simulink model "Nexonar_Navigation"  (R2018b)
settings: Solver=FixedStepDiscrete  StartTime=0.0  StopTime=0.1  RelTol=1e-3  EnableMultiTasking=on
libraries: commutil2 x12, c2833xlib x5, c280xlib x5, simulink x1, c2000lib x1
(part 1 of 2)
settings Model: ExtModeTrigDuration=8  Creator=User  LastModifiedBy=hengw
settings DataIOCC: LimitDataPoints=on  SaveFormat=Array  SaveOutput=off  SaveTime=off
settings OptimizationCC: DefaultUnderspecifiedDataType=single  ExpressionDepthLimit=2147483647  LifeSpan=1  MaxStackSize=512
settings DebuggingCC: UnderspecifiedInitializationDetection=Classic  MergeDetectMultiDrivingBlocksExec=none  SolverPrmCheckMsg=warning  StateNameClashWarn=warning  SFUnexpectedBacktrackingDiag=warning  SFNoUnconditionalDefaultTransitionDiag=warning  SFExecutionAtInitializationDiag=none
settings HardwareCC: ProdBitPerChar=16  ProdBitPerInt=16  ProdBitPerPointer=32  ProdBitPerSizeT=32  ProdBitPerPtrDiffT=32  ProdLargestAtomicInteger=Integer  ProdLargestAtomicFloat=None  ProdWordSize=16  ProdLongLongMode=on  ProdHWDeviceType=Texas Instruments->C2000  TargetBitPerChar=16  TargetBitPerInt=16  TargetLargestAtomicInteger=Integer  TargetIntDivRoundTo=Zero  TargetEndianess=LittleEndian  TargetWordSize=16  TargetHWDeviceType=Texas Instruments->C2000  ProdEqTarget=off
settings ModelReferenceCC: PropagateSignalLabelsOutOfModel=off
settings SFSimCC: SimCustomSourceCode="#include \"i2c_reset.c\""  SimCustomHeaderCode="#include \"i2c_reset.h\""  SimUseLocalCustomCode=off  MATLABDynamicMemAlloc=off
settings RTWCC: SystemTargetFile=ert.tlc  HardwareBoard=TI Delfino F2833x  TemplateMakefile=ert_default_tmf  RTWUseLocalCustomCode=off  RTWUseSimCustomCode=on  CustomSourceCode="#include \"i2c_reset.c\""  CustomHeaderCode="#include \"i2c_reset.h\""  Toolchain=Texas Instruments Code Composer Studio (C2000)
settings CodeAppCC: IgnoreCustomStorageClasses=off  CustomSymbolStrType=$N$R$M  StateflowObjectComments=on  InternalIdentifier=Classic
settings ERTTargetCC: CodeReplacementLibrary=TI C28x  MultiwordLength=2048  ParMdlRefBuildCompliant=off  CPPClassGenCompliant=off  ConvertIfToSwitch=off  SuppressUnreachableDefaultCases=off
settings ConfigComp: CovMetricSettings=dw  CovHtmlReporting=on  CovSaveCumulativeToWorkspaceVar=on  CovSaveSingleToWorkspaceVar=on  CovExternalEMLEnable=off  PSAutoStubLUT=on

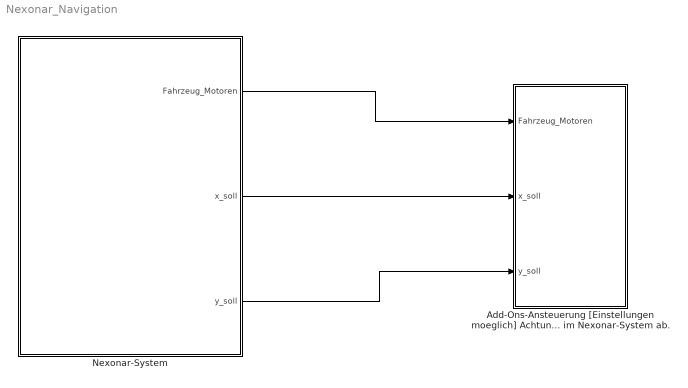
== system Nexonar_Navigation ==
  Add-Ons-Ansteuerung [Einstellungen moeglich] Achtung! Einige Einstellungswerte haengen von den Werten im Nexonar-System ab. : Subsystem
  Nexonar-System : Subsystem
  wires:
  Nexonar-System/2(x_soll) -> Add-Ons-Ansteuerung [Einstellungen moeglich] Achtung! Einige Einstellungswerte haengen von den Werten im Nexonar-System ab./2(x_soll)
  Nexonar-System/3(y_soll) -> Add-Ons-Ansteuerung [Einstellungen moeglich] Achtung! Einige Einstellungswerte haengen von den Werten im Nexonar-System ab./3(y_soll)
  Nexonar-System/1(Fahrzeug_Motoren) -> Add-Ons-Ansteuerung [Einstellungen moeglich] Achtung! Einige Einstellungswerte haengen von den Werten im Nexonar-System ab./1(Fahrzeug_Motoren)

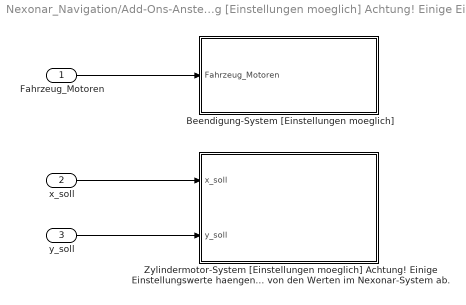
== system Nexonar_Navigation/Add-Ons-Ansteuerung [Einstellungen moeglich] Achtung! Einige Einstellungswerte haengen von den Werten im Nexonar-System ab. ==
  Fahrzeug_Motoren : Inport
  x_soll : Inport  Port=2
  y_soll : Inport  Port=3
  Beendigung-System [Einstellungen moeglich] : Subsystem
  Zylindermotor-System [Einstellungen moeglich] Achtung! Einige Einstellungswerte haengen von den Werten im Nexonar-System ab. : Subsystem
  wires:
  x_soll/1 -> Zylindermotor-System [Einstellungen moeglich] Achtung! Einige Einstellungswerte haengen von den Werten im Nexonar-System ab./1(x_soll)
  y_soll/1 -> Zylindermotor-System [Einstellungen moeglich] Achtung! Einige Einstellungswerte haengen von den Werten im Nexonar-System ab./2(y_soll)
  Fahrzeug_Motoren/1 -> Beendigung-System [Einstellungen moeglich]/1(Fahrzeug_Motoren)

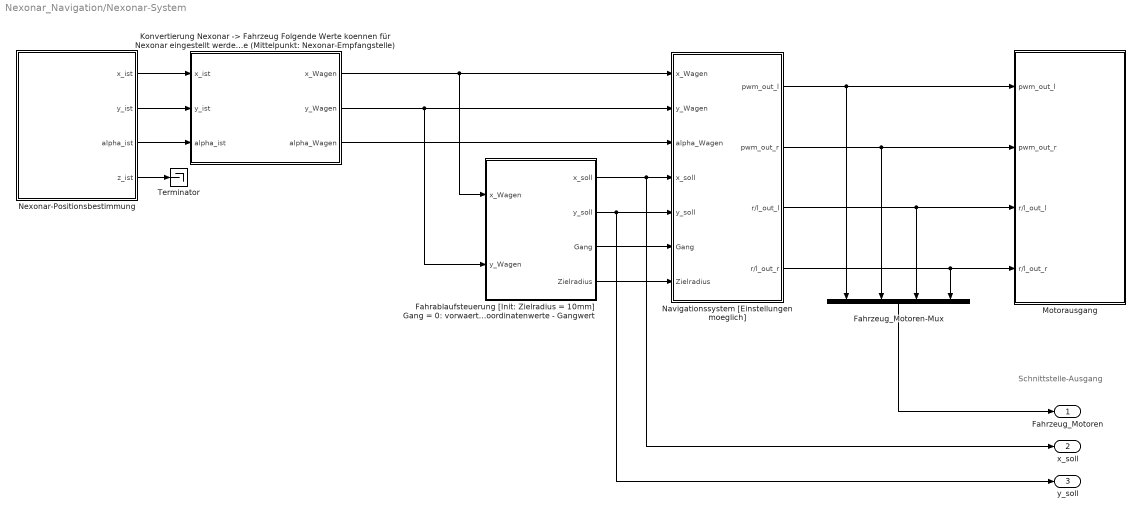
== system Nexonar_Navigation/Nexonar-System ==
  note: Schnittstelle-Ausgang
  Fahrablaufsteuerung [Init: Zielradius = 10mm] Gang = 0: vorwaerts Gang = 1: rueckwaerts Folgende Werte fuer den Ablauf sind einstellbar: - Zielkoordinatenwerte - Gangwert : Stateflow chart  TreatAsAtomicUnit=on
  Fahrzeug_Motoren-Mux : Mux
  "Konvertierung Nexonar -> Fahrzeug Folgende Werte koennen für Nexonar eingestellt werden: - r_Versatz_Nexo: Radialer Versatz des Nexonars zur Rotationsachse des Fahrzeugs - phi_Versatz_Nexo: Winkelversatz des Nexonars gegenüber der x-Achse (Mittelpunkt: Rotationspunkt des Fahrzeugs) - psi_Offset_Nexo: Winkelversatz des Nexonars gegenüber der x-Achse (Mittelpunkt: Nexonar-Empfangstelle)" : MATLAB Function  TreatAsAtomicUnit=on
  Motorausgang : Subsystem
  Navigationssystem [Einstellungen moeglich] : Subsystem  TreatAsAtomicUnit=on
  Nexonar-Positionsbestimmung : Subsystem
  Terminator : Terminator
  Fahrzeug_Motoren : Outport
  x_soll : Outport  Port=2
  y_soll : Outport  Port=3
  wires:
  Navigationssystem [Einstellungen moeglich]/3(r/l_out_l) -> Motorausgang/3(r/l_out_l), Fahrzeug_Motoren-Mux/3
  "Konvertierung Nexonar -> Fahrzeug Folgende Werte koennen für Nexonar eingestellt werden: - r_Versatz_Nexo: Radialer Versatz des Nexonars zur Rotationsachse des Fahrzeugs - phi_Versatz_Nexo: Winkelversatz des Nexonars gegenüber der x-Achse (Mittelpunkt: Rotationspunkt des Fahrzeugs) - psi_Offset_Nexo: Winkelversatz des Nexonars gegenüber der x-Achse (Mittelpunkt: Nexonar-Empfangstelle)"/2(y_Wagen) -> Fahrablaufsteuerung [Init: Zielradius = 10mm] Gang = 0: vorwaerts Gang = 1: rueckwaerts Folgende Werte fuer den Ablauf sind einstellbar: - Zielkoordinatenwerte - Gangwert/2(y_Wagen), Navigationssystem [Einstellungen moeglich]/2(y_Wagen)
  "Konvertierung Nexonar -> Fahrzeug Folgende Werte koennen für Nexonar eingestellt werden: - r_Versatz_Nexo: Radialer Versatz des Nexonars zur Rotationsachse des Fahrzeugs - phi_Versatz_Nexo: Winkelversatz des Nexonars gegenüber der x-Achse (Mittelpunkt: Rotationspunkt des Fahrzeugs) - psi_Offset_Nexo: Winkelversatz des Nexonars gegenüber der x-Achse (Mittelpunkt: Nexonar-Empfangstelle)"/1(x_Wagen) -> Fahrablaufsteuerung [Init: Zielradius = 10mm] Gang = 0: vorwaerts Gang = 1: rueckwaerts Folgende Werte fuer den Ablauf sind einstellbar: - Zielkoordinatenwerte - Gangwert/1(x_Wagen), Navigationssystem [Einstellungen moeglich]/1(x_Wagen)
  Nexonar-Positionsbestimmung/4(z_ist) -> Terminator/1
  Nexonar-Positionsbestimmung/1(x_ist) -> "Konvertierung Nexonar -> Fahrzeug Folgende Werte koennen für Nexonar eingestellt werden: - r_Versatz_Nexo: Radialer Versatz des Nexonars zur Rotationsachse des Fahrzeugs - phi_Versatz_Nexo: Winkelversatz des Nexonars gegenüber der x-Achse (Mittelpunkt: Rotationspunkt des Fahrzeugs) - psi_Offset_Nexo: Winkelversatz des Nexonars gegenüber der x-Achse (Mittelpunkt: Nexonar-Empfangstelle)"/1(x_ist)
  Fahrablaufsteuerung [Init: Zielradius = 10mm] Gang = 0: vorwaerts Gang = 1: rueckwaerts Folgende Werte fuer den Ablauf sind einstellbar: - Zielkoordinatenwerte - Gangwert/2(y_soll) -> y_soll/1, Navigationssystem [Einstellungen moeglich]/5(y_soll)
  Fahrablaufsteuerung [Init: Zielradius = 10mm] Gang = 0: vorwaerts Gang = 1: rueckwaerts Folgende Werte fuer den Ablauf sind einstellbar: - Zielkoordinatenwerte - Gangwert/1(x_soll) -> x_soll/1, Navigationssystem [Einstellungen moeglich]/4(x_soll)
  Navigationssystem [Einstellungen moeglich]/4(r/l_out_r) -> Motorausgang/4(r/l_out_r), Fahrzeug_Motoren-Mux/4
  Nexonar-Positionsbestimmung/3(alpha_ist) -> "Konvertierung Nexonar -> Fahrzeug Folgende Werte koennen für Nexonar eingestellt werden: - r_Versatz_Nexo: Radialer Versatz des Nexonars zur Rotationsachse des Fahrzeugs - phi_Versatz_Nexo: Winkelversatz des Nexonars gegenüber der x-Achse (Mittelpunkt: Rotationspunkt des Fahrzeugs) - psi_Offset_Nexo: Winkelversatz des Nexonars gegenüber der x-Achse (Mittelpunkt: Nexonar-Empfangstelle)"/3(alpha_ist)
  "Konvertierung Nexonar -> Fahrzeug Folgende Werte koennen für Nexonar eingestellt werden: - r_Versatz_Nexo: Radialer Versatz des Nexonars zur Rotationsachse des Fahrzeugs - phi_Versatz_Nexo: Winkelversatz des Nexonars gegenüber der x-Achse (Mittelpunkt: Rotationspunkt des Fahrzeugs) - psi_Offset_Nexo: Winkelversatz des Nexonars gegenüber der x-Achse (Mittelpunkt: Nexonar-Empfangstelle)"/3(alpha_Wagen) -> Navigationssystem [Einstellungen moeglich]/3(alpha_Wagen)
  Fahrablaufsteuerung [Init: Zielradius = 10mm] Gang = 0: vorwaerts Gang = 1: rueckwaerts Folgende Werte fuer den Ablauf sind einstellbar: - Zielkoordinatenwerte - Gangwert/3(Gang) -> Navigationssystem [Einstellungen moeglich]/6(Gang)
  Fahrablaufsteuerung [Init: Zielradius = 10mm] Gang = 0: vorwaerts Gang = 1: rueckwaerts Folgende Werte fuer den Ablauf sind einstellbar: - Zielkoordinatenwerte - Gangwert/4(Zielradius) -> Navigationssystem [Einstellungen moeglich]/7(Zielradius)
  Nexonar-Positionsbestimmung/2(y_ist) -> "Konvertierung Nexonar -> Fahrzeug Folgende Werte koennen für Nexonar eingestellt werden: - r_Versatz_Nexo: Radialer Versatz des Nexonars zur Rotationsachse des Fahrzeugs - phi_Versatz_Nexo: Winkelversatz des Nexonars gegenüber der x-Achse (Mittelpunkt: Rotationspunkt des Fahrzeugs) - psi_Offset_Nexo: Winkelversatz des Nexonars gegenüber der x-Achse (Mittelpunkt: Nexonar-Empfangstelle)"/2(y_ist)
  Fahrzeug_Motoren-Mux/1 -> Fahrzeug_Motoren/1
  Navigationssystem [Einstellungen moeglich]/1(pwm_out_l) -> Motorausgang/1(pwm_out_l), Fahrzeug_Motoren-Mux/1
  Navigationssystem [Einstellungen moeglich]/2(pwm_out_r) -> Motorausgang/2(pwm_out_r), Fahrzeug_Motoren-Mux/2

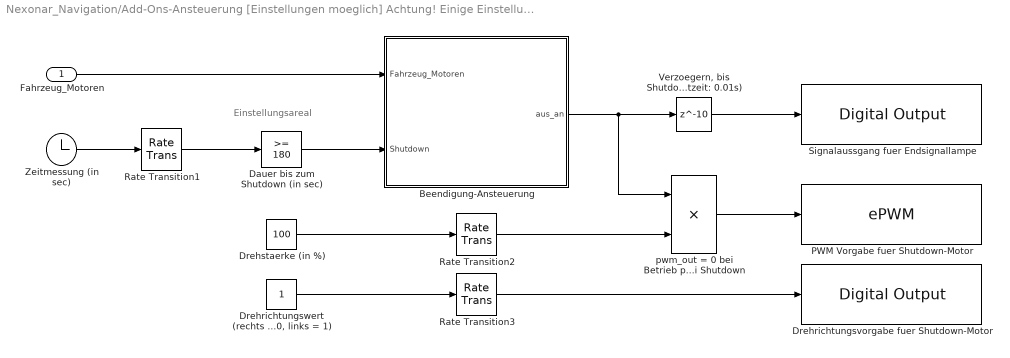
== system Nexonar_Navigation/Add-Ons-Ansteuerung [Einstellungen moeglich] Achtung! Einige Einstellungswerte haengen von den Werten im Nexonar-System ab./Beendigung-System [Einstellungen moeglich] ==
  note: Einstellungsareal
  Fahrzeug_Motoren : Inport
  Beendigung-Ansteuerung : Stateflow chart  TreatAsAtomicUnit=on
  Dauer bis zum Shutdown (in sec) : simulink/Logic and Bit Operations/Compare To Constant  relop=>=  const=180  OutDataTypeStr=boolean
  Drehrichtungsvorgabe fuer Shutdown-Motor : c2833xlib/Digital Output  GPIO_Number=GPIO8~GPIO15  GPIO_Bit0=off  GPIO_BIT0_Toggle=off  GPIO_Bit1=off  GPIO_BIT1_Toggle=off  GPIO_Bit2=off  GPIO_BIT2_Toggle=off  GPIO_Bit3=off  GPIO_BIT3_Toggle=off  GPIO_Bit4=off  GPIO_BIT4_Toggle=off  GPIO_Bit5=off  GPIO_BIT5_Toggle=off  GPIO_Bit6=off  GPIO_BIT6_Toggle=off  GPIO_Bit7=on  GPIO_BIT7_Toggle=off
      settings: SourceProductName=Embedded Coder Support Package for Texas Instruments C2000 Processors  SourceProductBaseCode=TIC2000
  "Drehrichtungswert (rechts = 0, links = 1)" : Constant
  Drehstaerke (in %) : Constant  Value=100
  "PWM Vorgabe fuer Shutdown-Motor " : c280xlib/ePWM  checkMode=off  useModule=ePWM5  periodUnits=Clock cycles  timerSource=Specify via dialog  timerPeriod_clk=64000  timerPeriod_sec=0.0001  tbshadow=Counter equals to zero  countingMode=Up  phaseActiveEnable=Disable  phaseDirection=Count down after sync  phaseActive=0  synchronizationEnable=off  synchronizationOption=Disable  clockPrescale=1  HSclockPrescale=1  ePWMxAStatus=off  CMPAUnits=Clock cycles  CMPASource=Specify via dialog  CMPAValue_per=50  CMPAValue_clk=32000  enCMPAshadow=Counter equals to zero  ePWMxAactionLogic1=Do nothing  ePWMxAactionLogic2=Clear  ePWMxAactionLogic3=Set  ePWMxAactionLogic4=Do nothing  ePWMxAactionLogic5=Do nothing  ePWMxAactionLogic6=Do nothing  ePWMxALoadMode=Load on counter equals to zero (CTR=Zero)  ePWMxACSFenable=off  ePWMxACSFvalue=Forcing disable  ePWMxASFreload=Zero  enHRPWM=off  HRPWM_LoadMode=Counter equals to zero (CTR=ZERO)  HRPWM_CTLMode=Phase control mode  HRPWM_EDGMode=Both edge  enSFO=on  ePWMxBStatus=on  CMPBUnits=Percentages  CMPBSource=Input port  CMPBValue_per=0  CMPBValue_clk=32000  enCMPBshadow=Counter equals to zero  ePWMxBactionLogic1=Do nothing  ePWMxBactionLogic2=Set  ePWMxBactionLogic3=Do nothing  ePWMxBactionLogic4=Do nothing  ePWMxBactionLogic5=Clear  ePWMxBactionLogic6=Do nothing  ePWMxBLoadMode=Load on counter equals to zero (CTR=Zero)  ePWMxBCSFenable=off  ePWMxBCSFvalue=Forcing disable  ePWMxBSFreload=Zero  enableDBePWMxA=off  enableDBePWMxB=off  DBpolarity=Active high (AH)  DBedgeDelay=Positive  DBSource_ePWMxA=ePWMxA  DBSource_ePWMxB=ePWMxA  DBperiodSource=Specify via dialog  REDperiod=0  FEDperiod=0  adcstartModuleA=off  adcrequestEventA=First event  adcstartEventA=Counter equals to zero (CTR=Zero)  adcstartModuleB=off  adcrequestEventB=First event  adcstartEventB=Counter equals to zero (CTR=Zero)  intEn=off  intPrd=First event  intSel=Counter equals to zero (CTR=Zero)  chopperEnable=off  chopperFrequency=1  chopperFirstwidth=1  chopperDuty=12.5%  tripZonesource=Specify via dialog  tzselOSHT1=off  tzselOSHT2=off  tzselOSHT3=off  tzselOSHT4=off  tzselOSHT5=off  tzselOSHT6=off  tzselCBC1=off  tzselCBC2=off  tzselCBC3=off  tzselCBC4=off  tzselCBC5=off  tzselCBC6=off  enTzOstIntr=off  enTzCbcIntr=off  ePWMxAforced=No action  ePWMxBforced=No action  timerPeriod=-1  ePWMxAValue=0  ePWMxBValue=0  tripZoneoption=One-shot trip (OSHT)
      settings: SourceProductName=Embedded Coder Support Package for Texas Instruments C2000 Processors  SourceProductBaseCode=TIC2000
  Rate Transition1 : RateTransition  OutPortSampleTime=0.01
  Rate Transition2 : RateTransition  OutPortSampleTime=0.01
  Rate Transition3 : RateTransition  OutPortSampleTime=0.01
  Signalaussgang fuer Endsignallampe : c2833xlib/Digital Output  GPIO_Number=GPIO56~GPIO63  GPIO_Bit0=off  GPIO_BIT0_Toggle=off  GPIO_Bit1=off  GPIO_BIT1_Toggle=off  GPIO_Bit2=on  GPIO_BIT2_Toggle=off  GPIO_Bit3=off  GPIO_BIT3_Toggle=off  GPIO_Bit4=off  GPIO_BIT4_Toggle=off  GPIO_Bit5=off  GPIO_BIT5_Toggle=off  GPIO_Bit6=off  GPIO_BIT6_Toggle=off  GPIO_Bit7=off  GPIO_BIT7_Toggle=off
      settings: SourceProductName=Embedded Coder Support Package for Texas Instruments C2000 Processors  SourceProductBaseCode=TIC2000
  "Verzoegern, bis Shutdown ausgefuehrt ist (Abtastzeit: 0.01s)" : Delay  DelayLength=10  InitialCondition=0
  Zeitmessung (in sec) : Clock
  pwm_out = 0 bei Betrieb pwm_out = Drehstaerke bei Shutdown : Product
  wires:
  Zeitmessung (in sec)/1 -> Rate Transition1/1
  pwm_out = 0 bei Betrieb pwm_out = Drehstaerke bei Shutdown/1 -> "PWM Vorgabe fuer Shutdown-Motor "/1
  "Drehrichtungswert (rechts = 0, links = 1)"/1 -> Rate Transition3/1
  Fahrzeug_Motoren/1 -> Beendigung-Ansteuerung/1(Fahrzeug_Motoren)
  Beendigung-Ansteuerung/1(aus_an) -> pwm_out = 0 bei Betrieb pwm_out = Drehstaerke bei Shutdown/1, "Verzoegern, bis Shutdown ausgefuehrt ist (Abtastzeit: 0.01s)"/1
  "Verzoegern, bis Shutdown ausgefuehrt ist (Abtastzeit: 0.01s)"/1 -> Signalaussgang fuer Endsignallampe/1
  Rate Transition3/1 -> Drehrichtungsvorgabe fuer Shutdown-Motor/1
  Dauer bis zum Shutdown (in sec)/1 -> Beendigung-Ansteuerung/2(Shutdown)
  Drehstaerke (in %)/1 -> Rate Transition2/1
  Rate Transition2/1 -> pwm_out = 0 bei Betrieb pwm_out = Drehstaerke bei Shutdown/2
  Rate Transition1/1 -> Dauer bis zum Shutdown (in sec)/1

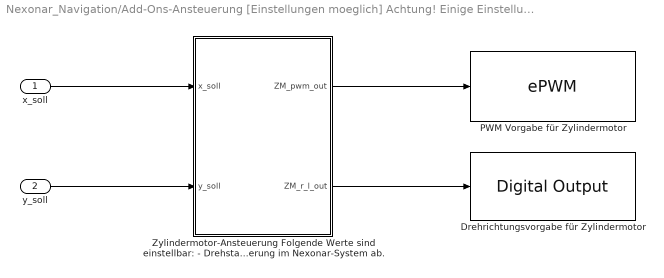
== system Nexonar_Navigation/Add-Ons-Ansteuerung [Einstellungen moeglich] Achtung! Einige Einstellungswerte haengen von den Werten im Nexonar-System ab./Zylindermotor-System [Einstellungen moeglich] Achtung! Einige Einstellungswerte haengen von den Werten im Nexonar-System ab. ==
  x_soll : Inport
  y_soll : Inport  Port=2
  Drehrichtungsvorgabe für Zylindermotor : c2833xlib/Digital Output  GPIO_Number=GPIO16~GPIO23  GPIO_Bit0=off  GPIO_BIT0_Toggle=off  GPIO_Bit1=on  GPIO_BIT1_Toggle=off  GPIO_Bit2=off  GPIO_BIT2_Toggle=off  GPIO_Bit3=off  GPIO_BIT3_Toggle=off  GPIO_Bit4=off  GPIO_BIT4_Toggle=off  GPIO_Bit5=off  GPIO_BIT5_Toggle=off  GPIO_Bit6=off  GPIO_BIT6_Toggle=off  GPIO_Bit7=off  GPIO_BIT7_Toggle=off
      settings: SourceProductName=Embedded Coder Support Package for Texas Instruments C2000 Processors  SourceProductBaseCode=TIC2000
  PWM Vorgabe für Zylindermotor : c280xlib/ePWM  checkMode=off  useModule=ePWM3  periodUnits=Clock cycles  timerSource=Specify via dialog  timerPeriod_clk=64000  timerPeriod_sec=0.0001  tbshadow=Counter equals to zero  countingMode=Up  phaseActiveEnable=Disable  phaseDirection=Count down after sync  phaseActive=0  synchronizationEnable=off  synchronizationOption=Disable  clockPrescale=1  HSclockPrescale=1  ePWMxAStatus=off  CMPAUnits=Clock cycles  CMPASource=Specify via dialog  CMPAValue_per=50  CMPAValue_clk=32000  enCMPAshadow=Counter equals to zero  ePWMxAactionLogic1=Do nothing  ePWMxAactionLogic2=Clear  ePWMxAactionLogic3=Set  ePWMxAactionLogic4=Do nothing  ePWMxAactionLogic5=Do nothing  ePWMxAactionLogic6=Do nothing  ePWMxALoadMode=Load on counter equals to zero (CTR=Zero)  ePWMxACSFenable=off  ePWMxACSFvalue=Forcing disable  ePWMxASFreload=Zero  enHRPWM=off  HRPWM_LoadMode=Counter equals to zero (CTR=ZERO)  HRPWM_CTLMode=Phase control mode  HRPWM_EDGMode=Both edge  enSFO=on  ePWMxBStatus=on  CMPBUnits=Percentages  CMPBSource=Input port  CMPBValue_per=0  CMPBValue_clk=32000  enCMPBshadow=Counter equals to zero  ePWMxBactionLogic1=Do nothing  ePWMxBactionLogic2=Set  ePWMxBactionLogic3=Do nothing  ePWMxBactionLogic4=Do nothing  ePWMxBactionLogic5=Clear  ePWMxBactionLogic6=Do nothing  ePWMxBLoadMode=Load on counter equals to zero (CTR=Zero)  ePWMxBCSFenable=off  ePWMxBCSFvalue=Forcing disable  ePWMxBSFreload=Zero  enableDBePWMxA=off  enableDBePWMxB=off  DBpolarity=Active high (AH)  DBedgeDelay=Positive  DBSource_ePWMxA=ePWMxA  DBSource_ePWMxB=ePWMxA  DBperiodSource=Specify via dialog  REDperiod=0  FEDperiod=0  adcstartModuleA=off  adcrequestEventA=First event  adcstartEventA=Counter equals to zero (CTR=Zero)  adcstartModuleB=off  adcrequestEventB=First event  adcstartEventB=Counter equals to zero (CTR=Zero)  intEn=off  intPrd=First event  intSel=Counter equals to zero (CTR=Zero)  chopperEnable=off  chopperFrequency=1  chopperFirstwidth=1  chopperDuty=12.5%  tripZonesource=Specify via dialog  tzselOSHT1=off  tzselOSHT2=off  tzselOSHT3=off  tzselOSHT4=off  tzselOSHT5=off  tzselOSHT6=off  tzselCBC1=off  tzselCBC2=off  tzselCBC3=off  tzselCBC4=off  tzselCBC5=off  tzselCBC6=off  enTzOstIntr=off  enTzCbcIntr=off  ePWMxAforced=No action  ePWMxBforced=No action  timerPeriod=-1  ePWMxAValue=0  ePWMxBValue=0  tripZoneoption=One-shot trip (OSHT)
      settings: SourceProductName=Embedded Coder Support Package for Texas Instruments C2000 Processors  SourceProductBaseCode=TIC2000
  "Zylindermotor-Ansteuerung Folgende Werte sind einstellbar: - Drehstaerke (in %) (-> ZM_pwm_out in \"Ausfuerung\") - Drehrichtung (rechts = 0, links = 1) (-> ZM_r_l_out in \"Init_und_Warten\") - Drehdauer (-> zwischen \"Ausfuehrung\" und \"Beendet\") - Ausfuehrungspunkt (in mm) [durch Wechsel der Soll-Position] (-> zwischen \"Init_und_Start\" und \"Ausfuehrung) Wichtig! Der Ausfuerungspunkt haengt von den EXAKTEN Soll-Werten aus der Fahrablaufsteuerung im Nexonar-System ab." : Stateflow chart  TreatAsAtomicUnit=on
  wires:
  "Zylindermotor-Ansteuerung Folgende Werte sind einstellbar: - Drehstaerke (in %) (-> ZM_pwm_out in \"Ausfuerung\") - Drehrichtung (rechts = 0, links = 1) (-> ZM_r_l_out in \"Init_und_Warten\") - Drehdauer (-> zwischen \"Ausfuehrung\" und \"Beendet\") - Ausfuehrungspunkt (in mm) [durch Wechsel der Soll-Position] (-> zwischen \"Init_und_Start\" und \"Ausfuehrung) Wichtig! Der Ausfuerungspunkt haengt von den EXAKTEN Soll-Werten aus der Fahrablaufsteuerung im Nexonar-System ab."/1(ZM_pwm_out) -> PWM Vorgabe für Zylindermotor/1
  "Zylindermotor-Ansteuerung Folgende Werte sind einstellbar: - Drehstaerke (in %) (-> ZM_pwm_out in \"Ausfuerung\") - Drehrichtung (rechts = 0, links = 1) (-> ZM_r_l_out in \"Init_und_Warten\") - Drehdauer (-> zwischen \"Ausfuehrung\" und \"Beendet\") - Ausfuehrungspunkt (in mm) [durch Wechsel der Soll-Position] (-> zwischen \"Init_und_Start\" und \"Ausfuehrung) Wichtig! Der Ausfuerungspunkt haengt von den EXAKTEN Soll-Werten aus der Fahrablaufsteuerung im Nexonar-System ab."/2(ZM_r_l_out) -> Drehrichtungsvorgabe für Zylindermotor/1
  y_soll/1 -> "Zylindermotor-Ansteuerung Folgende Werte sind einstellbar: - Drehstaerke (in %) (-> ZM_pwm_out in \"Ausfuerung\") - Drehrichtung (rechts = 0, links = 1) (-> ZM_r_l_out in \"Init_und_Warten\") - Drehdauer (-> zwischen \"Ausfuehrung\" und \"Beendet\") - Ausfuehrungspunkt (in mm) [durch Wechsel der Soll-Position] (-> zwischen \"Init_und_Start\" und \"Ausfuehrung) Wichtig! Der Ausfuerungspunkt haengt von den EXAKTEN Soll-Werten aus der Fahrablaufsteuerung im Nexonar-System ab."/2(y_soll)
  x_soll/1 -> "Zylindermotor-Ansteuerung Folgende Werte sind einstellbar: - Drehstaerke (in %) (-> ZM_pwm_out in \"Ausfuerung\") - Drehrichtung (rechts = 0, links = 1) (-> ZM_r_l_out in \"Init_und_Warten\") - Drehdauer (-> zwischen \"Ausfuehrung\" und \"Beendet\") - Ausfuehrungspunkt (in mm) [durch Wechsel der Soll-Position] (-> zwischen \"Init_und_Start\" und \"Ausfuehrung) Wichtig! Der Ausfuerungspunkt haengt von den EXAKTEN Soll-Werten aus der Fahrablaufsteuerung im Nexonar-System ab."/1(x_soll)

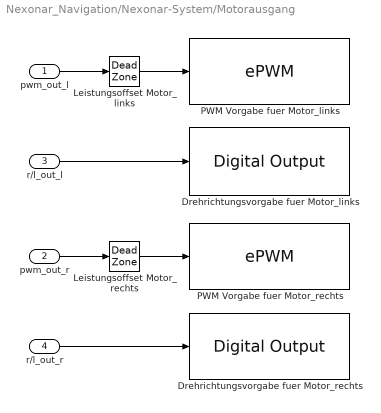
== system Nexonar_Navigation/Nexonar-System/Motorausgang ==
  pwm_out_l : Inport
  pwm_out_r : Inport  Port=2
  r/l_out_l : Inport  Port=3
  r/l_out_r : Inport  Port=4
  Drehrichtungsvorgabe fuer Motor_links : c2833xlib/Digital Output  GPIO_Number=GPIO16~GPIO23  GPIO_Bit0=off  GPIO_BIT0_Toggle=off  GPIO_Bit1=off  GPIO_BIT1_Toggle=off  GPIO_Bit2=off  GPIO_BIT2_Toggle=off  GPIO_Bit3=off  GPIO_BIT3_Toggle=off  GPIO_Bit4=on  GPIO_BIT4_Toggle=off  GPIO_Bit5=off  GPIO_BIT5_Toggle=off  GPIO_Bit6=off  GPIO_BIT6_Toggle=off  GPIO_Bit7=off  GPIO_BIT7_Toggle=off
      settings: SourceProductName=Embedded Coder Support Package for Texas Instruments C2000 Processors  SourceProductBaseCode=TIC2000
  Drehrichtungsvorgabe fuer Motor_rechts : c2833xlib/Digital Output  GPIO_Number=GPIO16~GPIO23  GPIO_Bit0=off  GPIO_BIT0_Toggle=off  GPIO_Bit1=off  GPIO_BIT1_Toggle=off  GPIO_Bit2=off  GPIO_BIT2_Toggle=off  GPIO_Bit3=off  GPIO_BIT3_Toggle=off  GPIO_Bit4=off  GPIO_BIT4_Toggle=off  GPIO_Bit5=on  GPIO_BIT5_Toggle=off  GPIO_Bit6=off  GPIO_BIT6_Toggle=off  GPIO_Bit7=off  GPIO_BIT7_Toggle=off
      settings: SourceProductName=Embedded Coder Support Package for Texas Instruments C2000 Processors  SourceProductBaseCode=TIC2000
  Leistungsoffset Motor_links : DeadZone  LowerValue=0  UpperValue=0  SaturateOnIntegerOverflow=on
  Leistungsoffset Motor_rechts : DeadZone  LowerValue=0  UpperValue=5  SaturateOnIntegerOverflow=on
  "PWM Vorgabe fuer Motor_links " : c280xlib/ePWM  checkMode=off  useModule=ePWM1  periodUnits=Clock cycles  timerSource=Specify via dialog  timerPeriod_clk=64000  timerPeriod_sec=0.0001  tbshadow=Counter equals to zero  countingMode=Up  phaseActiveEnable=Disable  phaseDirection=Count down after sync  phaseActive=0  synchronizationEnable=off  synchronizationOption=Disable  clockPrescale=1  HSclockPrescale=1  ePWMxAStatus=off  CMPAUnits=Clock cycles  CMPASource=Specify via dialog  CMPAValue_per=50  CMPAValue_clk=32000  enCMPAshadow=Counter equals to zero  ePWMxAactionLogic1=Do nothing  ePWMxAactionLogic2=Clear  ePWMxAactionLogic3=Set  ePWMxAactionLogic4=Do nothing  ePWMxAactionLogic5=Do nothing  ePWMxAactionLogic6=Do nothing  ePWMxALoadMode=Load on counter equals to zero (CTR=Zero)  ePWMxACSFenable=off  ePWMxACSFvalue=Forcing disable  ePWMxASFreload=Zero  enHRPWM=off  HRPWM_LoadMode=Counter equals to zero (CTR=ZERO)  HRPWM_CTLMode=Phase control mode  HRPWM_EDGMode=Both edge  enSFO=on  ePWMxBStatus=on  CMPBUnits=Percentages  CMPBSource=Input port  CMPBValue_per=0  CMPBValue_clk=32000  enCMPBshadow=Counter equals to zero  ePWMxBactionLogic1=Do nothing  ePWMxBactionLogic2=Set  ePWMxBactionLogic3=Do nothing  ePWMxBactionLogic4=Do nothing  ePWMxBactionLogic5=Clear  ePWMxBactionLogic6=Do nothing  ePWMxBLoadMode=Load on counter equals to zero (CTR=Zero)  ePWMxBCSFenable=off  ePWMxBCSFvalue=Forcing disable  ePWMxBSFreload=Zero  enableDBePWMxA=off  enableDBePWMxB=off  DBpolarity=Active high (AH)  DBedgeDelay=Positive  DBSource_ePWMxA=ePWMxA  DBSource_ePWMxB=ePWMxA  DBperiodSource=Specify via dialog  REDperiod=0  FEDperiod=0  adcstartModuleA=off  adcrequestEventA=First event  adcstartEventA=Counter equals to zero (CTR=Zero)  adcstartModuleB=off  adcrequestEventB=First event  adcstartEventB=Counter equals to zero (CTR=Zero)  intEn=off  intPrd=First event  intSel=Counter equals to zero (CTR=Zero)  chopperEnable=off  chopperFrequency=1  chopperFirstwidth=1  chopperDuty=12.5%  tripZonesource=Specify via dialog  tzselOSHT1=off  tzselOSHT2=off  tzselOSHT3=off  tzselOSHT4=off  tzselOSHT5=off  tzselOSHT6=off  tzselCBC1=off  tzselCBC2=off  tzselCBC3=off  tzselCBC4=off  tzselCBC5=off  tzselCBC6=off  enTzOstIntr=off  enTzCbcIntr=off  ePWMxAforced=No action  ePWMxBforced=No action  timerPeriod=-1  ePWMxAValue=0  ePWMxBValue=0  tripZoneoption=One-shot trip (OSHT)
      settings: SourceProductName=Embedded Coder Support Package for Texas Instruments C2000 Processors  SourceProductBaseCode=TIC2000
  PWM Vorgabe fuer Motor_rechts : c280xlib/ePWM  checkMode=off  useModule=ePWM2  periodUnits=Clock cycles  timerSource=Specify via dialog  timerPeriod_clk=64000  timerPeriod_sec=0.0001  tbshadow=Counter equals to zero  countingMode=Up  phaseActiveEnable=Disable  phaseDirection=Count down after sync  phaseActive=0  synchronizationEnable=off  synchronizationOption=Disable  clockPrescale=1  HSclockPrescale=1  ePWMxAStatus=off  CMPAUnits=Clock cycles  CMPASource=Specify via dialog  CMPAValue_per=50  CMPAValue_clk=32000  enCMPAshadow=Counter equals to zero  ePWMxAactionLogic1=Do nothing  ePWMxAactionLogic2=Clear  ePWMxAactionLogic3=Set  ePWMxAactionLogic4=Do nothing  ePWMxAactionLogic5=Do nothing  ePWMxAactionLogic6=Do nothing  ePWMxALoadMode=Load on counter equals to zero (CTR=Zero)  ePWMxACSFenable=off  ePWMxACSFvalue=Forcing disable  ePWMxASFreload=Zero  enHRPWM=off  HRPWM_LoadMode=Counter equals to zero (CTR=ZERO)  HRPWM_CTLMode=Phase control mode  HRPWM_EDGMode=Both edge  enSFO=on  ePWMxBStatus=on  CMPBUnits=Percentages  CMPBSource=Input port  CMPBValue_per=0  CMPBValue_clk=32000  enCMPBshadow=Counter equals to zero  ePWMxBactionLogic1=Do nothing  ePWMxBactionLogic2=Set  ePWMxBactionLogic3=Do nothing  ePWMxBactionLogic4=Do nothing  ePWMxBactionLogic5=Clear  ePWMxBactionLogic6=Do nothing  ePWMxBLoadMode=Load on counter equals to zero (CTR=Zero)  ePWMxBCSFenable=off  ePWMxBCSFvalue=Forcing disable  ePWMxBSFreload=Zero  enableDBePWMxA=off  enableDBePWMxB=off  DBpolarity=Active high (AH)  DBedgeDelay=Positive  DBSource_ePWMxA=ePWMxA  DBSource_ePWMxB=ePWMxA  DBperiodSource=Specify via dialog  REDperiod=0  FEDperiod=0  adcstartModuleA=off  adcrequestEventA=First event  adcstartEventA=Counter equals to zero (CTR=Zero)  adcstartModuleB=off  adcrequestEventB=First event  adcstartEventB=Counter equals to zero (CTR=Zero)  intEn=off  intPrd=First event  intSel=Counter equals to zero (CTR=Zero)  chopperEnable=off  chopperFrequency=1  chopperFirstwidth=1  chopperDuty=12.5%  tripZonesource=Specify via dialog  tzselOSHT1=off  tzselOSHT2=off  tzselOSHT3=off  tzselOSHT4=off  tzselOSHT5=off  tzselOSHT6=off  tzselCBC1=off  tzselCBC2=off  tzselCBC3=off  tzselCBC4=off  tzselCBC5=off  tzselCBC6=off  enTzOstIntr=off  enTzCbcIntr=off  ePWMxAforced=No action  ePWMxBforced=No action  timerPeriod=-1  ePWMxAValue=0  ePWMxBValue=0  tripZoneoption=One-shot trip (OSHT)
      settings: SourceProductName=Embedded Coder Support Package for Texas Instruments C2000 Processors  SourceProductBaseCode=TIC2000
  wires:
  pwm_out_l/1 -> Leistungsoffset Motor_links/1
  pwm_out_r/1 -> Leistungsoffset Motor_rechts/1
  r/l_out_l/1 -> Drehrichtungsvorgabe fuer Motor_links/1
  r/l_out_r/1 -> Drehrichtungsvorgabe fuer Motor_rechts/1
  Leistungsoffset Motor_links/1 -> "PWM Vorgabe fuer Motor_links "/1
  Leistungsoffset Motor_rechts/1 -> PWM Vorgabe fuer Motor_rechts/1

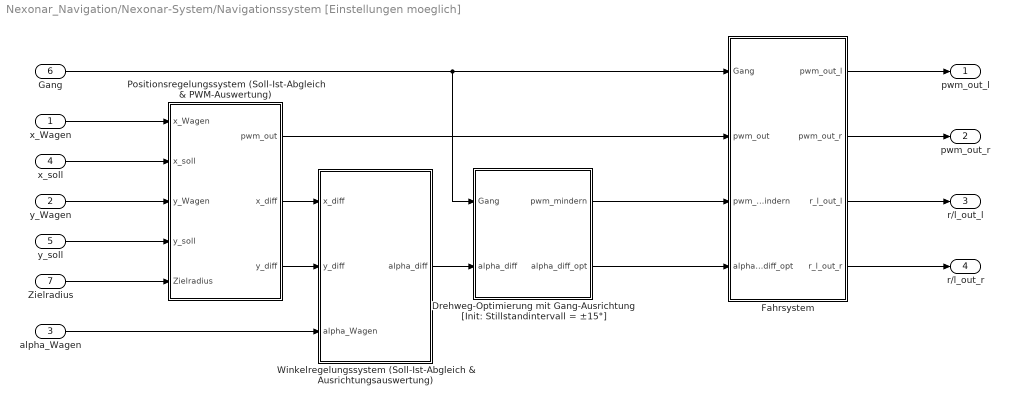
== system Nexonar_Navigation/Nexonar-System/Navigationssystem [Einstellungen moeglich] ==
  x_Wagen : Inport
  y_Wagen : Inport  Port=2
  alpha_Wagen : Inport  Port=3
  x_soll : Inport  Port=4
  y_soll : Inport  Port=5
  Gang : Inport  Port=6
  Zielradius : Inport  Port=7
  Drehweg-Optimierung mit Gang-Ausrichtung [Init: Stillstandintervall = ±15°] : Stateflow chart  TreatAsAtomicUnit=on
  Fahrsystem : Stateflow chart  TreatAsAtomicUnit=on
  Positionsregelungssystem (Soll-Ist-Abgleich & PWM-Auswertung) : Subsystem
  Winkelregelungssystem (Soll-Ist-Abgleich & Ausrichtungsauswertung) : Subsystem
  pwm_out_l : Outport
  pwm_out_r : Outport  Port=2
  r/l_out_l : Outport  Port=3
  r/l_out_r : Outport  Port=4
  wires:
  Positionsregelungssystem (Soll-Ist-Abgleich & PWM-Auswertung)/2(x_diff) -> Winkelregelungssystem (Soll-Ist-Abgleich & Ausrichtungsauswertung)/1(x_diff)
  y_soll/1 -> Positionsregelungssystem (Soll-Ist-Abgleich & PWM-Auswertung)/4(y_soll)
  y_Wagen/1 -> Positionsregelungssystem (Soll-Ist-Abgleich & PWM-Auswertung)/3(y_Wagen)
  Gang/1 -> Fahrsystem/1(Gang), Drehweg-Optimierung mit Gang-Ausrichtung [Init: Stillstandintervall = ±15°]/1(Gang)
  Positionsregelungssystem (Soll-Ist-Abgleich & PWM-Auswertung)/3(y_diff) -> Winkelregelungssystem (Soll-Ist-Abgleich & Ausrichtungsauswertung)/2(y_diff)
  x_Wagen/1 -> Positionsregelungssystem (Soll-Ist-Abgleich & PWM-Auswertung)/1(x_Wagen)
  x_soll/1 -> Positionsregelungssystem (Soll-Ist-Abgleich & PWM-Auswertung)/2(x_soll)
  alpha_Wagen/1 -> Winkelregelungssystem (Soll-Ist-Abgleich & Ausrichtungsauswertung)/3(alpha_Wagen)
  Fahrsystem/2(pwm_out_r) -> pwm_out_r/1
  Fahrsystem/4(r_l_out_r) -> r/l_out_r/1
  Fahrsystem/1(pwm_out_l) -> pwm_out_l/1
  Fahrsystem/3(r_l_out_l) -> r/l_out_l/1
  Winkelregelungssystem (Soll-Ist-Abgleich & Ausrichtungsauswertung)/1(alpha_diff) -> Drehweg-Optimierung mit Gang-Ausrichtung [Init: Stillstandintervall = ±15°]/2(alpha_diff)
  Drehweg-Optimierung mit Gang-Ausrichtung [Init: Stillstandintervall = ±15°]/2(alpha_diff_opt) -> Fahrsystem/4(alpha_diff_opt)
  Zielradius/1 -> Positionsregelungssystem (Soll-Ist-Abgleich & PWM-Auswertung)/5(Zielradius)
  Drehweg-Optimierung mit Gang-Ausrichtung [Init: Stillstandintervall = ±15°]/1(pwm_mindern) -> Fahrsystem/3(pwm_mindern)
  Positionsregelungssystem (Soll-Ist-Abgleich & PWM-Auswertung)/1(pwm_out) -> Fahrsystem/2(pwm_out)

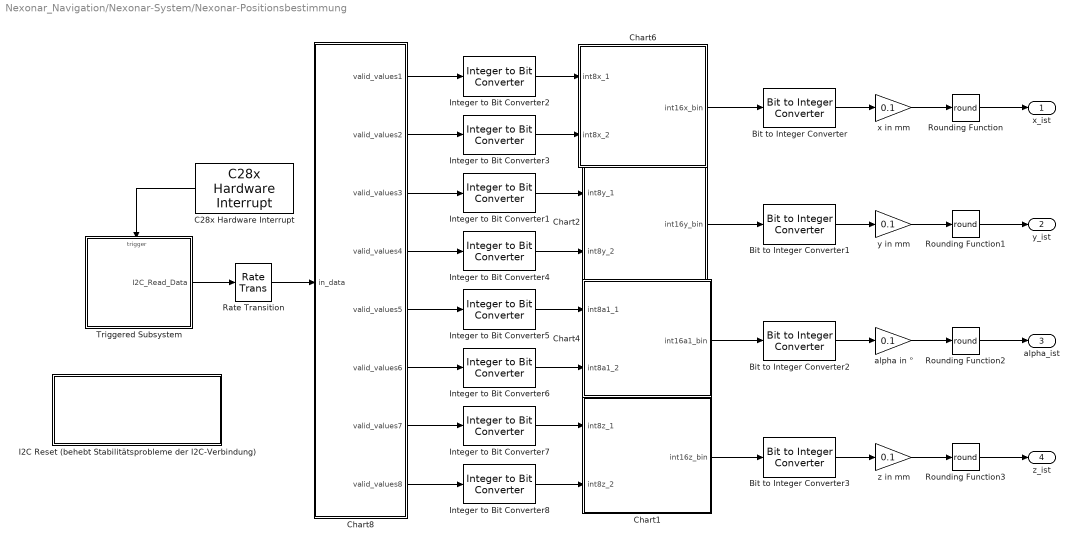
== system Nexonar_Navigation/Nexonar-System/Nexonar-Positionsbestimmung ==
  Bit to Integer Converter{,1..3} (4 alike) : commutil2/Bit to Integer Converter  nbits=16  bitOrder=MSB first  signedOutputValues=Signed  outDtype=Inherit via internal rule  outDtypeSigned=Inherit via internal rule
      settings: SourceProductName=Communications Toolbox
  C28x Hardware Interrupt : c2000lib/Scheduling/C28x Hardware Interrupt  irqnumbers=8  pienumbers=2  irqpriorities=30  irqpreempts=0  showinput=off  dspchiptype=C280X
      settings: SourceProductName=Embedded Coder Support Package for Texas Instruments C2000 Processors  SourceProductBaseCode=TIC2000
  Chart1 : Stateflow chart  TreatAsAtomicUnit=on
  Chart2 : Stateflow chart  TreatAsAtomicUnit=on
  Chart4 : Stateflow chart  TreatAsAtomicUnit=on
  Chart6 : Stateflow chart  TreatAsAtomicUnit=on
  Chart8 : Stateflow chart  TreatAsAtomicUnit=on
  I2C Reset (behebt Stabilitätsprobleme der I2C-Verbindung) : Subsystem
  Integer to Bit Converter{1..8} (8 alike) : commutil2/Integer to Bit Converter  nbits=8  signedInputValues=Unsigned  bitOrder=MSB first  outDtype=uint8
      settings: SourceProductName=Communications Toolbox
  Rate Transition : RateTransition  Deterministic=off  OutPortSampleTime=0.01
  Rounding Function{,1..3} (4 alike) : Rounding  Operator=round
  Triggered Subsystem : Subsystem  TreatAsAtomicUnit=on
  alpha in ° : Gain  Gain=0.1  OutDataTypeStr=double
  x in mm : Gain  Gain=0.1  OutDataTypeStr=double
  y in mm : Gain  Gain=0.1  OutDataTypeStr=double
  z in mm : Gain  Gain=0.1  OutDataTypeStr=double
  x_ist : Outport
  y_ist : Outport  Port=2
  alpha_ist : Outport  Port=3
  z_ist : Outport  Port=4
  wires:
  Integer to Bit Converter7/1 -> Chart1/1(int8z_1)
  Integer to Bit Converter8/1 -> Chart1/2(int8z_2)
  Chart8/7(valid_values7) -> Integer to Bit Converter7/1
  Chart8/8(valid_values8) -> Integer to Bit Converter8/1
  Triggered Subsystem/1(I2C_Read_Data) -> Rate Transition/1
  Chart1/1(int16z_bin) -> Bit to Integer Converter3/1
  Chart4/1(int16a1_bin) -> Bit to Integer Converter2/1
  Chart8/6(valid_values6) -> Integer to Bit Converter6/1
  Integer to Bit Converter6/1 -> Chart4/2(int8a1_2)
  Integer to Bit Converter5/1 -> Chart4/1(int8a1_1)
  Integer to Bit Converter4/1 -> Chart2/2(int8y_2)
  Integer to Bit Converter2/1 -> Chart6/1(int8x_1)
  Integer to Bit Converter1/1 -> Chart2/1(int8y_1)
  Chart6/1(int16x_bin) -> Bit to Integer Converter/1
  Integer to Bit Converter3/1 -> Chart6/2(int8x_2)
  Chart8/3(valid_values3) -> Integer to Bit Converter1/1
  Chart8/1(valid_values1) -> Integer to Bit Converter2/1
  Chart2/1(int16y_bin) -> Bit to Integer Converter1/1
  Chart8/4(valid_values4) -> Integer to Bit Converter4/1
  Chart8/2(valid_values2) -> Integer to Bit Converter3/1
  Chart8/5(valid_values5) -> Integer to Bit Converter5/1
  C28x Hardware Interrupt/1 -> Triggered Subsystem/Trigger
  Rate Transition/1 -> Chart8/1(in_data)
  x in mm/1 -> Rounding Function/1
  Bit to Integer Converter/1 -> x in mm/1
  Bit to Integer Converter1/1 -> y in mm/1
  y in mm/1 -> Rounding Function1/1
  Bit to Integer Converter3/1 -> z in mm/1
  z in mm/1 -> Rounding Function3/1
  Bit to Integer Converter2/1 -> alpha in °/1
  alpha in °/1 -> Rounding Function2/1
  Rounding Function/1 -> x_ist/1
  Rounding Function2/1 -> alpha_ist/1
  Rounding Function1/1 -> y_ist/1
  Rounding Function3/1 -> z_ist/1

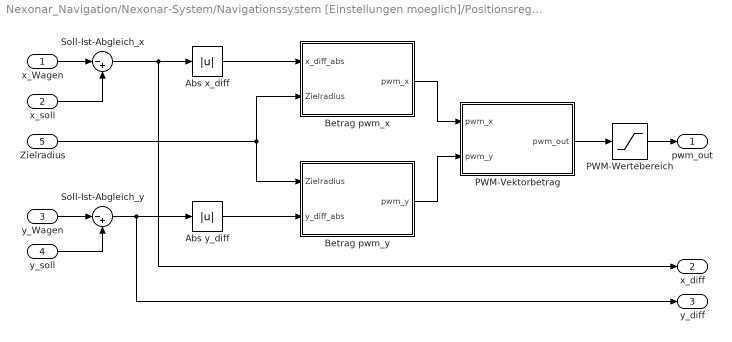
== system Nexonar_Navigation/Nexonar-System/Navigationssystem [Einstellungen moeglich]/Positionsregelungssystem (Soll-Ist-Abgleich & PWM-Auswertung) ==
  x_Wagen : Inport
  x_soll : Inport  Port=2
  y_Wagen : Inport  Port=3
  y_soll : Inport  Port=4
  Zielradius : Inport  Port=5
  Abs x_diff : Abs  SampleTime=0.01
  Abs y_diff : Abs  SampleTime=0.01
  Betrag pwm_x : MATLAB Function  TreatAsAtomicUnit=on  SystemSampleTime=0.01
  Betrag pwm_y : MATLAB Function  TreatAsAtomicUnit=on  SystemSampleTime=0.01
  PWM-Vektorbetrag : MATLAB Function  TreatAsAtomicUnit=on
  PWM-Wertebereich : Saturate  UpperLimit=100  LowerLimit=0
  Soll-Ist-Abgleich_x : Sum  Inputs=|-+  SampleTime=0.01
  Soll-Ist-Abgleich_y : Sum  Inputs=|-+  AccumDataTypeStr=double  SampleTime=0.01
  pwm_out : Outport
  x_diff : Outport  Port=2
  y_diff : Outport  Port=3
  wires:
  Soll-Ist-Abgleich_x/1 -> x_diff/1, Abs x_diff/1
  Abs x_diff/1 -> Betrag pwm_x/1(x_diff_abs)
  x_soll/1 -> Soll-Ist-Abgleich_x/2
  x_Wagen/1 -> Soll-Ist-Abgleich_x/1
  y_Wagen/1 -> Soll-Ist-Abgleich_y/1
  y_soll/1 -> Soll-Ist-Abgleich_y/2
  Soll-Ist-Abgleich_y/1 -> Abs y_diff/1, y_diff/1
  Abs y_diff/1 -> Betrag pwm_y/2(y_diff_abs)
  PWM-Wertebereich/1 -> pwm_out/1
  PWM-Vektorbetrag/1(pwm_out) -> PWM-Wertebereich/1
  Betrag pwm_x/1(pwm_x) -> PWM-Vektorbetrag/1(pwm_x)
  Betrag pwm_y/1(pwm_y) -> PWM-Vektorbetrag/2(pwm_y)
  Zielradius/1 -> Betrag pwm_y/1(Zielradius), Betrag pwm_x/2(Zielradius)

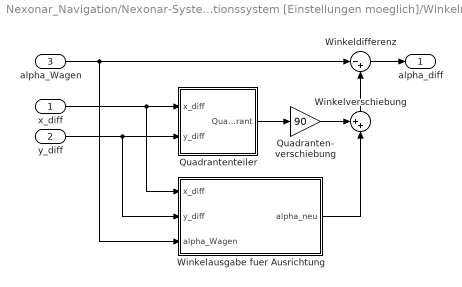
== system Nexonar_Navigation/Nexonar-System/Navigationssystem [Einstellungen moeglich]/Winkelregelungssystem (Soll-Ist-Abgleich & Ausrichtungsauswertung) ==
  x_diff : Inport
  y_diff : Inport  Port=2
  alpha_Wagen : Inport  Port=3
  Quadranten- verschiebung : Gain  Gain=90
  Quadrantenteiler : Stateflow chart  TreatAsAtomicUnit=on
  Winkelausgabe fuer Ausrichtung : Stateflow chart  TreatAsAtomicUnit=on
  Winkeldifferenz : Sum  Inputs=|-+
  Winkelverschiebung : Sum  Inputs=++|
  alpha_diff : Outport
  wires:
  alpha_Wagen/1 -> Winkelausgabe fuer Ausrichtung/3(alpha_Wagen), Winkeldifferenz/1
  y_diff/1 -> Winkelausgabe fuer Ausrichtung/2(y_diff), Quadrantenteiler/2(y_diff)
  Winkelausgabe fuer Ausrichtung/1(alpha_neu) -> Winkelverschiebung/2
  Winkelverschiebung/1 -> Winkeldifferenz/2
  x_diff/1 -> Winkelausgabe fuer Ausrichtung/1(x_diff), Quadrantenteiler/1(x_diff)
  Quadrantenteiler/1(Quadrant) -> Quadranten- verschiebung/1
  Winkeldifferenz/1 -> alpha_diff/1
  Quadranten- verschiebung/1 -> Winkelverschiebung/1

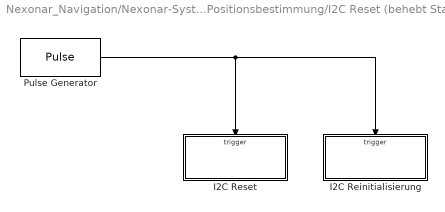
== system Nexonar_Navigation/Nexonar-System/Nexonar-Positionsbestimmung/I2C Reset (behebt Stabilitätsprobleme der I2C-Verbindung) ==
  I2C Reinitialisierung : Subsystem  TreatAsAtomicUnit=on
  I2C Reset : Subsystem  TreatAsAtomicUnit=on
  Pulse Generator : DiscretePulseGenerator  Period=250  SampleTime=0.01
  wires:
  Pulse Generator/1 -> I2C Reinitialisierung/Trigger, I2C Reset/Trigger

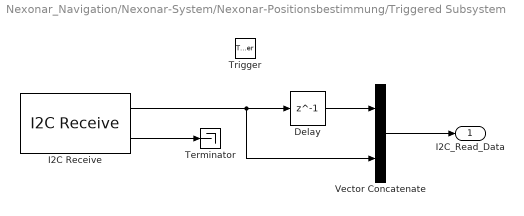
== system Nexonar_Navigation/Nexonar-System/Nexonar-Positionsbestimmung/Triggered Subsystem ==
  Trigger : TriggerPort  TriggerType=function-call  VariantControl=(inherit)
  Delay : Delay  DelayLength=1  InitialCondition=0
  I2C Receive : c280xlib/I2C Receive  selectModule=I2C_A  addrFormat=7-Bit addressing  saSource=Specify via dialog  SAR=80  bitCount=8  dataLength=10  initValue=0  NACK=on  STP=off  STR=on  sampleTime=-1  dataType=uint8
      settings: SourceProductName=Embedded Coder Support Package for Texas Instruments C2000 Processors  SourceProductBaseCode=TIC2000
  Terminator : Terminator
  Vector Concatenate : Concatenate
  I2C_Read_Data : Outport
  wires:
  I2C Receive/2 -> Terminator/1
  I2C Receive/1 -> Vector Concatenate/2, Delay/1
  Delay/1 -> Vector Concatenate/1
  Vector Concatenate/1 -> I2C_Read_Data/1

== system Nexonar_Navigation/Nexonar-System/Nexonar-Positionsbestimmung/I2C Reset (behebt Stabilitätsprobleme der I2C-Verbindung)/I2C Reinitialisierung ==
  Trigger : TriggerPort  TriggerType=falling  VariantControl=(inherit)
  I2C Reinitialisierung : MATLAB Function  TreatAsAtomicUnit=on

== system Nexonar_Navigation/Nexonar-System/Nexonar-Positionsbestimmung/I2C Reset (behebt Stabilitätsprobleme der I2C-Verbindung)/I2C Reset ==
  Trigger : TriggerPort  VariantControl=(inherit)
  I2C Reset : MATLAB Function  TreatAsAtomicUnit=on

== stateflow chart Nexonar_Navigation/Nexonar-System/Nexonar-Positionsbestimmung/Chart1 ==
  state Daten_einlesen
  state x0
  state x1_1
    entry: int16z_bin[0] = int8z_1[0];
    int16z_bin[1] = int8z_1[1];
    int16z_bin[2] = int8z_1[2];
    int16z_bin[3] = int8z_1[3];
    int16z_bin[4] = int8z_1[4];
    int16z_bin[5] = int8z_1[5]
    int16z_bin[6] = int8z_1[6];
    int16z_bin[7] = int8z_1[7];
    int16z_bin[8] = int8z_2[0];
    int16z_bin[9] = int8z_2[1];
    int16z_bin[10] = int8z_2[2];
    int16z_bin[11] = int8z_2[3];
    int16z_bin[12] = int8z_2[4];
    int16z_bin[13] = int8z_2[5]
    int16z_bin[14] = int8z_2[6];
    int16z_bin[15] = int8z_2[7];
  x0 -> Daten_einlesen
  (default) -> x0
  Daten_einlesen -> x1_1
  x1_1 -> Daten_einlesen
  data: int8z_1 input size=8; int8z_2 input size=8; int16z_bin output size=16 =0

== matlab function Nexonar_Navigation/Nexonar-System/Navigationssystem [Einstellungen moeglich]/Positionsregelungssystem (Soll-Ist-Abgleich & PWM-Auswertung)/PWM-Vektorbetrag ==
  data: pwm_x input; pwm_out output; pwm_y input
function pwm_out = fcn(pwm_x, pwm_y)

pwm_out = round(sqrt(pwm_x * pwm_x + pwm_y * pwm_y));

== stateflow chart Nexonar_Navigation/Add-Ons-Ansteuerung [Einstellungen moeglich] Achtung! Einige Einstellungswerte haengen von den Werten im Nexonar-System ab./Beendigung-System [Einstellungen moeglich]/Beendigung-Ansteuerung ==
  state Start_Warten
  state Aus_Zustand
    entry:
    aus_an = 0;
  state Anschalten
    entry:
    aus_an = 1;
  (default) -> Start_Warten
  Start_Warten -> Aus_Zustand
  Aus_Zustand -> Anschalten [order 1] : [Shutdown == 1]
  Aus_Zustand -> Anschalten [order 2] : [Fahrzeug_Motoren(1) == 0 && Fahrzeug_Motoren(2) == 0 ...
      | && Fahrzeug_Motoren(3) == Fahrzeug_Motoren(4)]
  data: aus_an output; Fahrzeug_Motoren input; Shutdown input

== matlab function Nexonar_Navigation/Nexonar-System/Konvertierung Nexonar -> Fahrzeug Folgende Werte koennen für Nexonar eingestellt werden: - r_Versatz_Nexo: Radialer Versatz des Nexonars zur Rotationsachse des Fahrzeugs - phi_Versatz_Nexo: Winkelversatz des Nexonars gegenüber der x-Achse (Mittelpunkt: Rotationspunkt des Fahrzeugs) - psi_Offset_Nexo: Winkelversatz des Nexonars gegenüber der x-Achse (Mittelpunkt: Nexonar-Empfangstelle) ==
  data: x_ist input; x_Wagen output; y_ist input; alpha_ist input; y_Wagen output; alpha_Wagen output
function [x_Wagen, y_Wagen, alpha_Wagen] = fcn(x_ist, y_ist, alpha_ist)

r_Versatz_Nexo = 2.5; % in mm
phi_Versatz_Nexo = 30; % in °
psi_Offset_Nexo = 15; % in 


alpha_Wagen = alpha_ist - psi_Offset_Nexo;
x_Wagen = x_ist - round(r_Versatz_Nexo * cos((phi_Versatz_Nexo+alpha_Wagen)*2*pi/360));
y_Wagen = y_ist - round(r_Versatz_Nexo * sin((phi_Versatz_Nexo+alpha_Wagen)*2*pi/360));

== stateflow chart Nexonar_Navigation/Nexonar-System/Fahrablaufsteuerung [Init: Zielradius = 10mm] Gang = 0: vorwaerts Gang = 1: rueckwaerts Folgende Werte fuer den Ablauf sind einstellbar: - Zielkoordinatenwerte - Gangwert ==
  state Sammeln1 [commented out]
    state Anfahrpunkt_1 [commented out]
      entry:
      x_soll = 1500;
      y_soll = 0;
    state Wechsel_1 [commented out]
      entry:
      Counter = Counter + 1;
    state Anfahrpunkt_2 [commented out]
      entry:
      x_soll = 1200;
      y_soll = 100;
    state Wechsel_2 [commented out]
      entry:
      Counter = Counter + 1;
    state Anfahrpunkt_3 [commented out]
      entry:
      x_soll = 1000;
      y_soll = 250;
    state Wechsel_3 [commented out]
      entry:
      Counter = Counter + 1;
    state Anfahrpunkt_4 [commented out]
      entry:
      x_soll = 940;
      y_soll = 650;
    state Wechsel_4 [commented out]
      entry:
      Counter = Counter + 1;
    state Anfahrpunkt_5 [commented out]
      entry:
      x_soll = 850;
      y_soll = 750;
    state Wechsel_5 [commented out]
      entry:
      Counter = Counter + 1;
    state Wechsel_10 [commented out]
      entry:
      Counter = Counter + 1;
    state Anfahrpunkt_6 [commented out]
      entry:
      x_soll = 600;
      y_soll = 825;
    state Anfahrpunkt_10 [commented out]
      entry:
      x_soll = 880;
      y_soll = 0;
    state Wechsel_6 [commented out]
      entry:
      Counter = Counter + 1;
    state Anfahrpunkt_7 [commented out]
      entry:
      x_soll = 500;
      y_soll = 825;
    state Wechsel_7 [commented out]
      entry:
      Counter = Counter + 1;
    state Anfahrpunkt_8 [commented out]
      entry:
      x_soll = 325;
      y_soll = 725;
    state Wechsel_8 [commented out]
      entry:
      Counter = Counter + 1;
    state Anfahrpunkt_9 [commented out]
      entry:
      x_soll = 400;
      y_soll = 300;
    state Wechsel_9 [commented out]
      entry:
      Counter = Counter + 1;
    state Anfahrpunkt_11 [commented out]
      entry:
      x_soll = 600;
      y_soll = 0;
    state Wechsel_11 [commented out]
      entry:
      Counter = Counter + 1;
    state Anfahrpunkt_12 [commented out]
      entry:
      x_soll = 900;
      y_soll = 0;
    state Wechsel_12 [commented out]
      entry:
      Counter = Counter + 1;
    state Anfahrpunkt_13 [commented out]
      entry:
      x_soll = 1200;
      y_soll = 0;
    state Wechsel_13 [commented out]
      entry:
      Counter = Counter + 1;
    state Anfahrpunkt_14 [commented out]
      entry:
      x_soll = 1420;
      y_soll = -100;
    state Wechsel_14 [commented out]
      entry:
      Counter = Counter + 1;
    (default) -> Anfahrpunkt_1 [commented out] : {Counter = 0}
    Anfahrpunkt_1 -> Sammeln1.Wechsel_1 [commented out] : [abs(x_soll - x_Wagen) <= Zielradius && abs(y_soll - y_Wagen) <= Zielradius]
    Sammeln1.Wechsel_1 -> Anfahrpunkt_2 [commented out]
    Anfahrpunkt_2 -> Sammeln1.Wechsel_2 [commented out] : [abs(x_soll - x_Wagen) <= Zielradius && abs(y_soll - y_Wagen) <= Zielradius]
    Sammeln1.Wechsel_2 -> Anfahrpunkt_3 [commented out]
    Anfahrpunkt_3 -> Sammeln1.Wechsel_3 [commented out] : [abs(x_soll - x_Wagen) <= Zielradius && abs(y_soll - y_Wagen) <= Zielradius]
    Sammeln1.Wechsel_3 -> Anfahrpunkt_4 [commented out]
    Wechsel_10 -> Anfahrpunkt_4 [commented out]
    Anfahrpunkt_4 -> Wechsel_4 [commented out] : [abs(x_soll - x_Wagen) <= Zielradius && abs(y_soll - y_Wagen) <= Zielradius]
    Wechsel_4 -> Anfahrpunkt_5 [commented out]
    Anfahrpunkt_5 -> Wechsel_5 [commented out] : [abs(x_soll - x_Wagen) <= Zielradius && abs(y_soll - y_Wagen) <= Zielradius]
    Wechsel_5 -> Anfahrpunkt_6 [commented out]
    Anfahrpunkt_10 -> Wechsel_10 [commented out] : [abs(x_soll - x_Wagen) <= Zielradius && abs(y_soll - y_Wagen) <= Zielradius]
    Anfahrpunkt_6 -> Wechsel_6 [commented out] : [abs(x_soll - x_Wagen) <= Zielradius && abs(y_soll - y_Wagen) <= Zielradius]
    Wechsel_9 -> Anfahrpunkt_10 [commented out] : [Counter == 9]
    Wechsel_6 -> Anfahrpunkt_7 [commented out]
    Anfahrpunkt_7 -> Wechsel_7 [commented out] : [abs(x_soll - x_Wagen) <= Zielradius && abs(y_soll - y_Wagen) <= Zielradius]
    Wechsel_7 -> Anfahrpunkt_8 [commented out]
    Anfahrpunkt_8 -> Wechsel_8 [commented out] : [abs(x_soll - x_Wagen) <= Zielradius && abs(y_soll - y_Wagen) <= Zielradius]
    Wechsel_8 -> Anfahrpunkt_9 [commented out]
    Anfahrpunkt_9 -> Wechsel_9 [commented out] : [abs(x_soll - x_Wagen) <= Zielradius && abs(y_soll - y_Wagen) <= Zielradius]
    Wechsel_9 -> Anfahrpunkt_11 [commented out]
    Anfahrpunkt_11 -> Wechsel_11 [commented out] : [abs(x_soll - x_Wagen) <= Zielradius && abs(y_soll - y_Wagen) <= Zielradius]
    Wechsel_11 -> Anfahrpunkt_12 [commented out]
    Anfahrpunkt_12 -> Wechsel_12 [commented out] : [abs(x_soll - x_Wagen) <= Zielradius && abs(y_soll - y_Wagen) <= Zielradius]
    Wechsel_12 -> Anfahrpunkt_13 [commented out]
    Anfahrpunkt_13 -> Wechsel_13 [commented out] : [abs(x_soll - x_Wagen) <= Zielradius && abs(y_soll - y_Wagen) <= Zielradius]
    Wechsel_13 -> Sammeln1.Anfahrpunkt_14 [commented out]
    Sammeln1.Anfahrpunkt_14 -> Sammeln1.Wechsel_14 [commented out] : [abs(x_soll - x_Wagen) <= Zielradius && abs(y_soll - y_Wagen) <= Zielradius]
  state Parken
    state Parken_1
      entry:
      x_soll = 1420;
      y_soll = -50;
    state Wechsel_1
      entry:
      Counter = Counter + 1;
    state Parken_2
      entry:
      x_soll = 1620;
      y_soll = -135;
    state Wechsel_2
      entry:
      Counter = Counter + 1;
    state Parken_3
      entry:
      x_soll = 1640;
      y_soll = -131;
    state Wechsel_3
      entry:
      Counter = Counter + 1;
    (default) -> Parken_1 : {Counter = 0}
    Parken_1 -> Parken.Wechsel_1 : [abs(x_soll - x_Wagen) <= Zielradius && abs(y_soll - y_Wagen) <= Zielradius]
    Parken.Wechsel_1 -> Parken_2
    Parken_2 -> Parken.Wechsel_2 : [abs(x_soll - x_Wagen) <= Zielradius && abs(y_soll - y_Wagen) <= Zielradius]
    Parken.Wechsel_2 -> Parken_3
    Parken_3 -> Parken.Wechsel_3 : [abs(x_soll - x_Wagen) <= Zielradius && abs(y_soll - y_Wagen) <= Zielradius]
  state Uebergabe
    state Uebergabepunkt_x_Richtung
      entry:
      x_soll = 1414;
      y_soll = y_least;
    state Wechsel_1
      entry:
      Counter = Counter + 1;
    state Uebergabepunkt_y_Richtung
      entry:
      x_soll = x_least;
      y_soll = 5;
    state Warten_Uebergabe
    state Wechsel_2
      entry:
      Counter = Counter + 1;
    (default) -> Uebergabepunkt_x_Richtung : {Counter = 0}
    Uebergabepunkt_x_Richtung -> Uebergabe.Wechsel_1 : [abs(x_soll - x_Wagen) <= Zielradius && abs(y_soll - y_Wagen) <= Zielradius]
        | {x_least = x_soll; y_least = y_soll;}
    Uebergabe.Wechsel_1 -> Uebergabepunkt_y_Richtung
    Uebergabepunkt_y_Richtung -> Warten_Uebergabe : [abs(x_soll - x_Wagen) <= Zielradius && abs(y_soll - y_Wagen) <= Zielradius]
    Warten_Uebergabe -> Uebergabe.Wechsel_2 : [after(1,sec)]
  state Start_Einstellung_Init
    entry:
    Zielradius = 10;
  state Sammeln
    state Anfahrpunkt_14
      entry:
      x_soll = 1420;
      y_soll = -100;
    state Wechsel_14
      entry:
      Counter = Counter + 1;
    (default) -> Sammeln.Anfahrpunkt_14 : {Counter = 0}
    Sammeln.Anfahrpunkt_14 -> Sammeln.Wechsel_14 : [abs(x_soll - x_Wagen) <= Zielradius && abs(y_soll - y_Wagen) <= Zielradius]
  state Ende
  Sammeln1 -> ? [commented out] : [Counter == 20]
      | {Gang = 1;
      | x_least = x_soll;
      | y_least = y_soll;}
  (default) -> Start_Einstellung_Init
  Sammeln -> Uebergabe : [Counter == 1]
      | {Gang = 1;
      | x_least = x_soll;
      | y_least = y_soll;}
  Uebergabe -> Parken : [Counter == 2]{Gang = 0}
  Start_Einstellung_Init -> Sammeln : {Gang = 0}
  Parken -> Ende : [Counter == 3]
  data: x_soll output; y_soll output; x_Wagen input; y_Wagen input; Counter local; x_least local; y_least local; Gang output; Zielradius output

== stateflow chart Nexonar_Navigation/Add-Ons-Ansteuerung [Einstellungen moeglich] Achtung! Einige Einstellungswerte haengen von den Werten im Nexonar-System ab./Zylindermotor-System [Einstellungen moeglich] Achtung! Einige Einstellungswerte haengen von den Werten im Nexonar-System ab./Zylindermotor-Ansteuerung Folgende Werte sind einstellbar: - Drehstaerke (in %) (-> ZM_pwm_out in "Ausfuerung") - Drehrichtung (rechts = 0, links = 1) (-> ZM_r_l_out in "Init_und_Warten") - Drehdauer (-> zwischen "Ausfuehrung" und "Beendet") - Ausfuehrungspunkt (in mm) [durch Wechsel der Soll-Position] (-> zwischen "Init_und_Start" und "Ausfuehrung) Wichtig! Der Ausfuerungspunkt haengt von den EXAKTEN Soll-Werten aus der Fahrablaufsteuerung im Nexonar-System ab. ==
  state Init_und_Warten
    entry:
    ZM_pwm_out = 0;
    ZM_r_l_out = 1;
  state Ausfuehrung
    entry:
    ZM_pwm_out = 50;
  state Beendet
    entry:
    ZM_pwm_out = 0;
  Init_und_Warten -> Ausfuehrung : [x_soll == 1200 && y_soll == 0]
  (default) -> Init_und_Warten
  Ausfuehrung -> Beendet : [after(0.1,sec)]
  data: ZM_pwm_out output; ZM_r_l_out output; x_soll input; y_soll input
